simulink library "Lib_LongPRACH"  (R2023b)
settings: Solver=VariableStepAuto  StartTime=0.0  StopTime=10.0  RelTol=1e-3
values from neighbouring files (symbols this model uses):
  prach = waveconfig.PRACH.Config    [hNRPRACHWaveformGenerator.m]
undefined symbols (not defined in the file or in its folder): AdvDSPBChannelOutDisplay, AdvDSPBDMemDisplay, AdvDSPBInDisplay, AdvDSPBOutDisplay, dpoly, dspba, dspba_ChannelInVis, dspba_ChannelOutVis, dspba_internal_get_channel_ports, evalAionMaskParam, latency, latencyCorrection, NTxAnts, primtype, UseDontCare, value
libraries: DSPBAPrim x553, DSPBABase x32, DSPBAFilters x24, DSPBAControl x18, DSPBAModelBus x8, DSPBAWaveformSynth x4, DspbAdvFftLibrary x2, DSPBAUtilities x2
(part 6 of 8)

== system Lib_LongPRACH/prach_wrap/SYM_SELECT/Zero_insertion/Zeropad_rear ==
  valid_in : Inport
  chin : Inport  Port=2
  datain : Inport  Port=3
  And : DSPBAPrim/And  primtype=and  nInputs=2  nOutputs=1  omode=Inherit via internal rule  otype=sfix(16)  scale=2^-15  rndmethod=Unbiased  factor=1  satmethod=Symmetric  shift_vec=[0 1 2 -1]  value=0  inPortNames=[' '; ' '; ' '; ' '; ' '; ' '; ' '; ' '; ' '; ' '; ' '; ' '; ' '; ' '; ' '; ' '; ]  outPortNames=[' ']  dspbaimage=dspba_prim.svg  text=fprintf('&');  style=Optimised  visibilities=8+2  version=20211007
  Const3 : DSPBAPrim/Const  primtype=const  nInputs=0  nOutputs=1  omode=Inherit via internal rule  otype=sfix(16)  scale=2^-15  rndmethod=Unbiased  factor=1  satmethod=Symmetric  shift_vec=[0 1 2 -1]  value=0  inPortNames=['+'; '+';]  outPortNames=[' ']  dspbaimage=dspba_prim.svg  text=fprintf('%s', num2str(value));  style=Optimised  visibilities=8 + 1024 + 2^18 + 2^20  floatPrecision=float32_m23  warnSaturation=on  version=20211007  SampleTime=inf
  Mux1 : DSPBAPrim/Mux  primtype=mux  nInputs=evalAionMaskParam(gcb,'value',1)+1  nOutputs=1  omode=Inherit via internal rule  otype=sfix(16)  scale=2^-15  rndmethod=Unbiased  factor=1  satmethod=Symmetric  shift_vec=[0 1 2 -1]  value=2  inPortNames=['s '; 'd0'; 'd1'; 'd2'; 'd3'; 'd4'; 'd5'; 'd6'; 'd7'; 'd8'; 'd9';]  outPortNames=[' ']  dspbaimage=dspba_prim_tall.svg  text=fprintf('%s', primtype);  style=Optimised  visibilities=1032  version=20211007
  Not : DSPBAPrim/Not  primtype=not  nInputs=1  nOutputs=1  omode=Inherit via internal rule  otype=sfix(16)  scale=2^-15  rndmethod=Unbiased  factor=1  satmethod=Symmetric  shift_vec=[0 1 2 -1]  value=0  inPortNames=[' '; ' ';]  outPortNames=[' ']  dspbaimage=dspba_prim.svg  text=fprintf('~');  style=Optimised  visibilities=8  version=20211007
  Or : DSPBAPrim/Or  primtype=or  nInputs=2  nOutputs=1  omode=Inherit via internal rule  otype=sfix(16)  scale=2^-15  rndmethod=Unbiased  factor=1  satmethod=Symmetric  shift_vec=[0 1 2 -1]  value=0  inPortNames=[' '; ' '; ' '; ' '; ' '; ' '; ' '; ' '; ' '; ' '; ' '; ' '; ' '; ' '; ' '; ' '; ]  outPortNames=[' ']  dspbaimage=dspba_prim.svg  text=fprintf('|');  style=Optimised  visibilities=8+2  version=20211007
  SampleDelay2 : DSPBAPrim/SampleDelay  primtype=sampdelay  nInputs=1  nOutputs=1  omode=Inherit via internal rule  otype=sfix(16)  scale=2^-15  rndmethod=Unbiased  factor=1  satmethod=Symmetric  shift_vec=[0 1 2 -1]  floatPrecision=float32_m23  value=ZeroPadRear  inPortNames=[' '; ' ';]  outPortNames=[' ']  dspbaimage=dspba_prim.svg  text=dpoly(1, eye(1,value+1), 'z')  style=Optimised  visibilities=8 + 2^11 + 2^18 + 2^19  flexible=off  slackgroup=0  augmented=0  version=20211007  advOptions=[]
  valid_out : Outport
  "chout " : Outport  Port=2
  dataout : Outport  Port=3
  wires:
  Const3/1 -> Mux1/3
  Mux1/1 -> dataout/1
  Not/1 -> And/2
  Or/1 -> valid_out/1
  datain/1 -> Mux1/2
  chin/1 -> "chout "/1
  SampleDelay2/1 -> And/1, Or/2
  valid_in/1 -> Not/1, Or/1, SampleDelay2/1
  And/1 -> Mux1/1

== system Lib_LongPRACH/Longprach_C_M_plane/LongPRACH_core/CP_REMOVAL/RemoveCP5/syncgen ==
  In1 : Inport
  CmpEQ : DSPBAPrim/CmpEQ  primtype=cmpeq  nInputs=2  nOutputs=1  omode=boolean  otype=sfix(16)  scale=2^-15  rndmethod=Unbiased  factor=1  satmethod=Symmetric  shift_vec=[0 1 2 -1]  value=0  inPortNames=[' '; ' ';]  outPortNames=[' ']  dspbaimage=dspba_prim.svg  text=fprintf('==');  style=Optimised  visibilities=0  advOptions=[]  version=20211007
  Const2 : DSPBAPrim/Const  primtype=const  nInputs=0  nOutputs=1  omode=Inherit via internal rule  otype=sfix(16)  scale=2^-15  rndmethod=Unbiased  factor=1  satmethod=Symmetric  shift_vec=[0 1 2 -1]  value=10  inPortNames=['+'; '+';]  outPortNames=[' ']  dspbaimage=dspba_prim.svg  text=fprintf('%s', num2str(value));  style=Optimised  visibilities=8 + 1024 + 2^18 + 2^20  floatPrecision=float32_m23  warnSaturation=on  version=20211007  SampleTime=inf
  Const3 : DSPBAPrim/Const  primtype=const  nInputs=0  nOutputs=1  omode=Inherit via internal rule  otype=sfix(16)  scale=2^-15  rndmethod=Unbiased  factor=1  satmethod=Symmetric  shift_vec=[0 1 2 -1]  value=4  inPortNames=['+'; '+';]  outPortNames=[' ']  dspbaimage=dspba_prim.svg  text=fprintf('%s', num2str(value));  style=Optimised  visibilities=8 + 1024 + 2^18 + 2^20  floatPrecision=float32_m23  warnSaturation=on  version=20211007  SampleTime=inf
  StretchPulse : DSPBAControl/StretchPulse
  q : Outport
  wires:
  Const2/1 -> CmpEQ/2
  CmpEQ/1 -> StretchPulse/1
  Const3/1 -> StretchPulse/2
  StretchPulse/1 -> q/1
  In1/1 -> CmpEQ/1

== system Lib_LongPRACH/Longprach_C_M_plane/LongPRACH_core/DECIMATION1/Stage1/Filt_DEC_by_3_stage1 ==
  din : Inport
  vin : Inport  Port=2
  cin : Inport  Port=3
  Complex to Real-Imag : ComplexToRealImag
  Const1 : DSPBAPrim/Const  primtype=const  nInputs=0  nOutputs=1  omode=Inherit via back propagation  otype=ufix(8)  scale=2^0  rndmethod=Unbiased  factor=1  satmethod=Symmetric  shift_vec=[0 1 2 -1]  value=deimator_shift  inPortNames=['+'; '+';]  outPortNames=[' ']  dspbaimage=dspba_prim.svg  text=fprintf('%s', num2str(value));  style=Optimised  visibilities=8 + 1024  floatPrecision=float32_m23  warnSaturation=on  version=20211007  SampleTime=inf
  Const6 : DSPBAPrim/Const  primtype=const  nInputs=0  nOutputs=1  omode=Inherit via back propagation  otype=ufix(8)  scale=2^0  rndmethod=Unbiased  factor=1  satmethod=Symmetric  shift_vec=[0 1 2 -1]  value=deimator_shift  inPortNames=['+'; '+';]  outPortNames=[' ']  dspbaimage=dspba_prim.svg  text=fprintf('%s', num2str(value));  style=Optimised  visibilities=8 + 1024  floatPrecision=float32_m23  warnSaturation=on  version=20211007  SampleTime=inf
  DecimatingFIR1 : DSPBAFilters/DecimatingFIR  nInputRate=prach.MaxSampleRate  decim=3  nchan=prach.no_of_chan  symmetry=Symmetrical  coef=b_decimator1  addr=MMoffset.decby3_st2  rwmode=Constant  nband=Use All Taps  exposebus=off  latency=26  version=20090407  recon=off  MM=[0,1,2,3,4,5,6,7,8,9,10,11,12,13,14,15]  resetrezero=off  sharecoef=auto  simulationMode=Standard
  DecimatingFIR2 : DSPBAFilters/DecimatingFIR  nInputRate=prach.MaxSampleRate  decim=3  nchan=prach.no_of_chan  symmetry=Symmetrical  coef=b_decimator1  addr=MMoffset.decby3_st2  rwmode=Constant  nband=Use All Taps  exposebus=off  latency=26  version=20090407  recon=off  MM=[0,1,2,3,4,5,6,7,8,9,10,11,12,13,14,15]  resetrezero=off  sharecoef=auto  simulationMode=Standard
  Real-Imag to Complex : RealImagToComplex
  Scale : DSPBABase/Scale  otype=sfix(16)  scale=2^-15  rndmethod=Biased  factor=decimator_gain1  satmethod=Symmetric  shift_vec=0  latency=5  simulationMode=Use Global Value  version=20130807
  Scale1 : DSPBABase/Scale  otype=sfix(16)  scale=2^-15  rndmethod=Biased  factor=decimator_gain1  satmethod=Symmetric  shift_vec=0  latency=5  simulationMode=Use Global Value  version=20130807
  Terminator : Terminator
  Terminator1 : Terminator
  To Workspace3 : ToWorkspace  VariableName=dec_dout_stage1  SampleTime=-1
  To Workspace4 : ToWorkspace  VariableName=dec_vout_stage1  SampleTime=-1
  dout : Outport  VectorParamsAs1DForOutWhenUnconnected=off
  vout : Outport  Port=2  VectorParamsAs1DForOutWhenUnconnected=off
  cout : Outport  Port=3  VectorParamsAs1DForOutWhenUnconnected=off
  wires:
  Scale/3 -> cout/1
  DecimatingFIR2/2 -> Scale/2
  vin/1 -> DecimatingFIR1/2, DecimatingFIR2/2
  DecimatingFIR2/3 -> Scale/3
  Scale/2 -> To Workspace4/1, vout/1
  Scale/4 -> Terminator/1
  cin/1 -> DecimatingFIR1/3, DecimatingFIR2/3
  Const6/1 -> Scale/4
  DecimatingFIR2/1 -> Scale/1
  din/1 -> Complex to Real-Imag/1
  Complex to Real-Imag/1 -> DecimatingFIR2/1
  Complex to Real-Imag/2 -> DecimatingFIR1/1
  Scale1/1 -> Real-Imag to Complex/2
  DecimatingFIR1/3 -> Scale1/3
  Scale1/4 -> Terminator1/1
  DecimatingFIR1/1 -> Scale1/1
  DecimatingFIR1/2 -> Scale1/2
  Const1/1 -> Scale1/4
  Real-Imag to Complex/1 -> To Workspace3/1, dout/1
  Scale/1 -> Real-Imag to Complex/1

== system Lib_LongPRACH/Longprach_C_M_plane/LongPRACH_core/DECIMATION1/Stage1/filt_flush_in ==
  note: 1 0 0 0
  data_in : Inport
  valid_in : Inport  Port=2
  ch_in : Inport  Port=3
  flush_en : Inport  Port=4
  ChannelIn : DSPBAPrim/ChannelIn  primtype=channelin  nInputs=dspba_internal_get_channel_ports(gcb)  nOutputs=dspba_internal_get_channel_ports(gcb)  omode=Inherit via internal rule  otype=sfix(16)  scale=2^-15  rndmethod=Unbiased  factor=1  satmethod=Symmetric  shift_vec=[0 1 2 -1]  value=2  inPortNames=['v'; 'c'; '0'; '1'; '2'; '3'; '4'; '5'; '6'; '7'; '8'; '9'; 'A'; 'B'; 'D'; 'E'; 'F'; 'G'; 'H'; 'I'; 'J'; 'K'; 'L'; 'M'; 'N'; 'O'; 'P'; 'Q'; 'R'; 'S'; 'T'; 'U'; 'W'; 'X'; 'Y'; 'Z']  outPortNames=['v'; 'c'; '0'; '1'; '2'; '3'; '4'; '5'; '6'; '7'; '8'; '9'; 'A'; 'B'; 'D'; 'E'; 'F'; 'G'; 'H'; 'I'; 'J'; 'K'; 'L'; 'M'; 'N'; 'O'; 'P'; 'Q'; 'R'; 'S'; 'T'; 'U'; 'W'; 'X'; 'Y'; 'Z']  dspbaimage=dspba_prim_channel_tall.svg  text=fprintf('In');  style=Optimised  dataSignals=2  foldingEnabled=off  channels=1  sampleRate=200  packetBeginPresent=off  packetBeginEnabled=off  visibilities=dspba_ChannelInVis(gcb)  latencyCorrection=0  scheduleOrigin=on  version=20211214
  ChannelOut : DSPBAPrim/ChannelOut  primtype=channelout  nInputs=dspba_internal_get_channel_ports(gcb)  nOutputs=dspba_internal_get_channel_ports(gcb)  omode=Inherit via internal rule  otype=sfix(16)  scale=2^-15  rndmethod=Unbiased  factor=1  satmethod=Symmetric  shift_vec=[0 1 2 -1]  value=1  inPortNames=['v'; 'c'; '0'; '1'; '2'; '3'; '4'; '5'; '6'; '7'; '8'; '9'; 'A'; 'B'; 'D'; 'E'; 'F'; 'G'; 'H'; 'I'; 'J'; 'K'; 'L'; 'M'; 'N'; 'O'; 'P'; 'Q'; 'R'; 'S'; 'T'; 'U'; 'W'; 'X'; 'Y'; 'Z']  outPortNames=['v'; 'c'; '0'; '1'; '2'; '3'; '4'; '5'; '6'; '7'; '8'; '9'; 'A'; 'B'; 'D'; 'E'; 'F'; 'G'; 'H'; 'I'; 'J'; 'K'; 'L'; 'M'; 'N'; 'O'; 'P'; 'Q'; 'R'; 'S'; 'T'; 'U'; 'W'; 'X'; 'Y'; 'Z']  dspbaimage=dspba_prim_channel_tall.svg  text=fprintf('Out%s', AdvDSPBChannelOutDisplay(latency));  style=Optimised  dataSignals=1  foldingEnabled=off  channels=1  sampleRate=200  packetBeginPresent=off  packetBeginEnabled=off  visibilities=dspba_ChannelOutVis(gcb)  latency=1  latencyCorrection=0  version=20211214
  Const1 : DSPBAPrim/Const  primtype=const  nInputs=0  nOutputs=1  omode=Inherit via internal rule  otype=sfix(16)  scale=2^-15  rndmethod=Unbiased  factor=1  satmethod=Symmetric  shift_vec=[0 1 2 -1]  value=0  inPortNames=['+'; '+';]  outPortNames=[' ']  dspbaimage=dspba_prim.svg  text=fprintf('%s', num2str(value));  style=Optimised  visibilities=8 + 1024 + 2^18 + 2^20  floatPrecision=float32_m23  warnSaturation=on  version=20211007  SampleTime=inf
  Mux : DSPBAPrim/Mux  primtype=mux  nInputs=evalAionMaskParam(gcb,'value',1)+1  nOutputs=1  omode=Inherit via internal rule  otype=sfix(16)  scale=2^-15  rndmethod=Unbiased  factor=1  satmethod=Symmetric  shift_vec=[0 1 2 -1]  value=2  inPortNames=['s '; 'd0'; 'd1'; 'd2'; 'd3'; 'd4'; 'd5'; 'd6'; 'd7'; 'd8'; 'd9';]  outPortNames=[' ']  dspbaimage=dspba_prim_tall.svg  text=fprintf('%s', primtype);  style=Optimised  visibilities=1032  version=20211007
  Mux1 : DSPBAPrim/Mux  primtype=mux  nInputs=evalAionMaskParam(gcb,'value',1)+1  nOutputs=1  omode=Inherit via internal rule  otype=sfix(16)  scale=2^-15  rndmethod=Unbiased  factor=1  satmethod=Symmetric  shift_vec=[0 1 2 -1]  value=2  inPortNames=['s '; 'd0'; 'd1'; 'd2'; 'd3'; 'd4'; 'd5'; 'd6'; 'd7'; 'd8'; 'd9';]  outPortNames=[' ']  dspbaimage=dspba_prim_tall.svg  text=fprintf('%s', primtype);  style=Optimised  visibilities=1032  version=20211007
  Mux2 : DSPBAPrim/Mux  primtype=mux  nInputs=evalAionMaskParam(gcb,'value',1)+1  nOutputs=1  omode=Inherit via internal rule  otype=sfix(16)  scale=2^-15  rndmethod=Unbiased  factor=1  satmethod=Symmetric  shift_vec=[0 1 2 -1]  value=2  inPortNames=['s '; 'd0'; 'd1'; 'd2'; 'd3'; 'd4'; 'd5'; 'd6'; 'd7'; 'd8'; 'd9';]  outPortNames=[' ']  dspbaimage=dspba_prim_tall.svg  text=fprintf('%s', primtype);  style=Optimised  visibilities=1032  version=20211007
  SynthesisInfo : DSPBAPrim/SynthesisInfo  primtype=synthinfo  nInputs=0  nOutputs=0  omode=Inherit via internal rule  otype=sfix(16)  scale=2^-15  rndmethod=Truncate  factor=1  satmethod=Symmetric  shift_vec=[0 1 2 -1]  value=99  inPortNames=[' '; ' ';]  outPortNames=[' ']  dspbaimage=dspba_prim_ctrl.jpg  text=fprintf('Style=%s', style);  style=Scheduled  visibilities=2^17+2^18+2^19+2^20+2^21+2^22+2^23+2^24  constraintPair=None  constraintRelation=>  constraintLimit=2  modelRefSign=+  modelRef=''  showSchedule=off  simulationMode=Use Global Value  resetMinimization=Conditional - On for ChannelIn/Out only  version=20220106
  ch_pulse : Subsystem
  data_out : Outport
  valid_out : Outport  Port=2
  ch_out : Outport  Port=3
  wires:
  Mux/1 -> ChannelOut/1
  ChannelOut/1 -> valid_out/1
  Mux2/1 -> ChannelOut/3
  flush_en/1 -> ChannelIn/4
  Const1/1 -> Mux2/3
  ChannelOut/3 -> data_out/1
  ChannelIn/2 -> Mux1/2
  ChannelOut/2 -> ch_out/1
  ch_in/1 -> ChannelIn/2
  ChannelIn/1 -> Mux/2
  valid_in/1 -> ChannelIn/1
  ChannelIn/3 -> Mux2/2
  ChannelIn/4 -> Mux2/1, ch_pulse/1(In1), Mux1/1, Mux/1, Mux/3
  Mux1/1 -> ChannelOut/2
  data_in/1 -> ChannelIn/3
  ch_pulse/1(Out1) -> Mux1/3

== system Lib_LongPRACH/Longprach_C_M_plane/LongPRACH_core/DECIMATION1/Stage2/Filt_DEC_by_2_stage2 ==
  din : Inport
  vin : Inport  Port=2
  cin : Inport  Port=3
  Complex to Real-Imag : ComplexToRealImag
  Const1 : DSPBAPrim/Const  primtype=const  nInputs=0  nOutputs=1  omode=Inherit via back propagation  otype=ufix(8)  scale=2^0  rndmethod=Unbiased  factor=1  satmethod=Symmetric  shift_vec=[0 1 2 -1]  value=deimator_shift  inPortNames=['+'; '+';]  outPortNames=[' ']  dspbaimage=dspba_prim.svg  text=fprintf('%s', num2str(value));  style=Optimised  visibilities=8 + 1024  floatPrecision=float32_m23  warnSaturation=on  version=20211007  SampleTime=inf
  Const6 : DSPBAPrim/Const  primtype=const  nInputs=0  nOutputs=1  omode=Inherit via back propagation  otype=ufix(8)  scale=2^0  rndmethod=Unbiased  factor=1  satmethod=Symmetric  shift_vec=[0 1 2 -1]  value=deimator_shift  inPortNames=['+'; '+';]  outPortNames=[' ']  dspbaimage=dspba_prim.svg  text=fprintf('%s', num2str(value));  style=Optimised  visibilities=8 + 1024  floatPrecision=float32_m23  warnSaturation=on  version=20211007  SampleTime=inf
  DecimatingFIR : DSPBAFilters/DecimatingFIR  nInputRate=prach.MaxSampleRate/3  decim=2  nchan=prach.no_of_chan  symmetry=Symmetrical  coef=b_decimator2  addr=MMoffset.HBcoef3  rwmode=Constant  nband=Use All Taps  exposebus=off  latency=34  version=20090407  recon=off  MM=[0,1,2,3,4,5,6,7,8,9,10,11,12,13,14,15]  resetrezero=off  sharecoef=auto  simulationMode=Standard
  DecimatingFIR1 : DSPBAFilters/DecimatingFIR  nInputRate=prach.MaxSampleRate/3  decim=2  nchan=prach.no_of_chan  symmetry=Symmetrical  coef=b_decimator2  addr=MMoffset.HBcoef3  rwmode=Constant  nband=Use All Taps  exposebus=off  latency=34  version=20090407  recon=off  MM=[0,1,2,3,4,5,6,7,8,9,10,11,12,13,14,15]  resetrezero=off  sharecoef=auto  simulationMode=Standard
  Real-Imag to Complex : RealImagToComplex
  Scale : DSPBABase/Scale  otype=sfix(16)  scale=2^-15  rndmethod=Biased  factor=decimator_gain2  satmethod=Symmetric  shift_vec=0  latency=5  simulationMode=Use Global Value  version=20130807
  Scale1 : DSPBABase/Scale  otype=sfix(16)  scale=2^-15  rndmethod=Biased  factor=decimator_gain2  satmethod=Symmetric  shift_vec=0  latency=5  simulationMode=Use Global Value  version=20130807
  Terminator{,1..3} (4 alike) : Terminator
  To Workspace3 : ToWorkspace  VariableName=dec_dout_stage2  SampleTime=-1
  To Workspace4 : ToWorkspace  VariableName=dec_vout_stage2  SampleTime=-1
  dout : Outport  VectorParamsAs1DForOutWhenUnconnected=off
  vout : Outport  Port=2  VectorParamsAs1DForOutWhenUnconnected=off
  cout : Outport  Port=3  VectorParamsAs1DForOutWhenUnconnected=off
  wires:
  DecimatingFIR/1 -> Scale/1
  Const6/1 -> Scale/4
  cin/1 -> DecimatingFIR1/3, DecimatingFIR/3
  Scale/4 -> Terminator/1
  DecimatingFIR/3 -> Scale/3
  vin/1 -> DecimatingFIR1/2, DecimatingFIR/2
  DecimatingFIR/2 -> Scale/2
  Scale/3 -> cout/1
  din/1 -> Complex to Real-Imag/1
  Complex to Real-Imag/1 -> DecimatingFIR/1
  Complex to Real-Imag/2 -> DecimatingFIR1/1
  DecimatingFIR1/1 -> Scale1/1
  DecimatingFIR1/3 -> Scale1/3
  Scale1/1 -> Real-Imag to Complex/2
  DecimatingFIR1/2 -> Scale1/2
  Const1/1 -> Scale1/4
  Scale1/4 -> Terminator1/1
  Scale/1 -> Real-Imag to Complex/1
  Scale1/2 -> Terminator2/1
  Scale1/3 -> Terminator3/1
  Scale/2 -> To Workspace4/1, vout/1
  Real-Imag to Complex/1 -> To Workspace3/1, dout/1

== system Lib_LongPRACH/Longprach_C_M_plane/LongPRACH_core/DECIMATION1/Stage3/Filt_DEC_by_2_stage3 ==
  din : Inport
  vin : Inport  Port=2
  cin : Inport  Port=3
  Complex to Real-Imag : ComplexToRealImag
  Const1 : DSPBAPrim/Const  primtype=const  nInputs=0  nOutputs=1  omode=Inherit via back propagation  otype=ufix(8)  scale=2^0  rndmethod=Unbiased  factor=1  satmethod=Symmetric  shift_vec=[0 1 2 -1]  value=deimator_shift  inPortNames=['+'; '+';]  outPortNames=[' ']  dspbaimage=dspba_prim.svg  text=fprintf('%s', num2str(value));  style=Optimised  visibilities=8 + 1024  floatPrecision=float32_m23  warnSaturation=on  version=20211007  SampleTime=inf
  Const6 : DSPBAPrim/Const  primtype=const  nInputs=0  nOutputs=1  omode=Inherit via back propagation  otype=ufix(8)  scale=2^0  rndmethod=Unbiased  factor=1  satmethod=Symmetric  shift_vec=[0 1 2 -1]  value=deimator_shift  inPortNames=['+'; '+';]  outPortNames=[' ']  dspbaimage=dspba_prim.svg  text=fprintf('%s', num2str(value));  style=Optimised  visibilities=8 + 1024  floatPrecision=float32_m23  warnSaturation=on  version=20211007  SampleTime=inf
  DecimatingFIR : DSPBAFilters/DecimatingFIR  nInputRate=prach.MaxSampleRate/(3*2)  decim=2  nchan=prach.no_of_chan  symmetry=Symmetrical  coef=b_decimator3  addr=MMoffset.HBcoef3  rwmode=Constant  nband=Use All Taps  exposebus=off  latency=46  version=20090407  recon=off  MM=[0,1,2,3,4,5,6,7,8,9,10,11,12,13,14,15]  resetrezero=off  sharecoef=auto  simulationMode=Standard
  DecimatingFIR1 : DSPBAFilters/DecimatingFIR  nInputRate=prach.MaxSampleRate/(3*2)  decim=2  nchan=prach.no_of_chan  symmetry=Symmetrical  coef=b_decimator3  addr=MMoffset.HBcoef3  rwmode=Constant  nband=Use All Taps  exposebus=off  latency=46  version=20090407  recon=off  MM=[0,1,2,3,4,5,6,7,8,9,10,11,12,13,14,15]  resetrezero=off  sharecoef=auto  simulationMode=Standard
  Real-Imag to Complex : RealImagToComplex
  Scale : DSPBABase/Scale  otype=sfix(16)  scale=2^-15  rndmethod=Biased  factor=decimator_gain3  satmethod=Symmetric  shift_vec=0  latency=5  simulationMode=Use Global Value  version=20130807
  Scale1 : DSPBABase/Scale  otype=sfix(16)  scale=2^-15  rndmethod=Biased  factor=decimator_gain3  satmethod=Symmetric  shift_vec=0  latency=5  simulationMode=Use Global Value  version=20130807
  Terminator{,1..3} (4 alike) : Terminator
  To Workspace3 : ToWorkspace  VariableName=dec_dout_stage3  SampleTime=-1
  To Workspace4 : ToWorkspace  VariableName=dec_vout_stage3  SampleTime=-1
  dout : Outport  VectorParamsAs1DForOutWhenUnconnected=off
  vout : Outport  Port=2  VectorParamsAs1DForOutWhenUnconnected=off
  cout : Outport  Port=3  VectorParamsAs1DForOutWhenUnconnected=off
  wires:
  DecimatingFIR/1 -> Scale/1
  Const6/1 -> Scale/4
  cin/1 -> DecimatingFIR1/3, DecimatingFIR/3
  Scale/4 -> Terminator/1
  DecimatingFIR/3 -> Scale/3
  vin/1 -> DecimatingFIR1/2, DecimatingFIR/2
  DecimatingFIR/2 -> Scale/2
  Scale/3 -> cout/1
  din/1 -> Complex to Real-Imag/1
  Complex to Real-Imag/1 -> DecimatingFIR/1
  Complex to Real-Imag/2 -> DecimatingFIR1/1
  DecimatingFIR1/1 -> Scale1/1
  DecimatingFIR1/3 -> Scale1/3
  Scale1/1 -> Real-Imag to Complex/2
  DecimatingFIR1/2 -> Scale1/2
  Const1/1 -> Scale1/4
  Scale1/4 -> Terminator1/1
  Scale/1 -> Real-Imag to Complex/1
  Scale1/2 -> Terminator2/1
  Scale1/3 -> Terminator3/1
  Scale/2 -> To Workspace4/1, vout/1
  Real-Imag to Complex/1 -> To Workspace3/1, dout/1

== system Lib_LongPRACH/Longprach_C_M_plane/LongPRACH_core/DECIMATION1/Stage5/Filt_DEC_by_2_stage5 ==
  din : Inport
  vin : Inport  Port=2
  cin : Inport  Port=3
  Complex to Real-Imag : ComplexToRealImag
  Const1 : DSPBAPrim/Const  primtype=const  nInputs=0  nOutputs=1  omode=Inherit via back propagation  otype=ufix(8)  scale=2^0  rndmethod=Unbiased  factor=1  satmethod=Symmetric  shift_vec=[0 1 2 -1]  value=deimator_shift  inPortNames=['+'; '+';]  outPortNames=[' ']  dspbaimage=dspba_prim.svg  text=fprintf('%s', num2str(value));  style=Optimised  visibilities=8 + 1024  floatPrecision=float32_m23  warnSaturation=on  version=20211007  SampleTime=inf
  Const6 : DSPBAPrim/Const  primtype=const  nInputs=0  nOutputs=1  omode=Inherit via back propagation  otype=ufix(8)  scale=2^0  rndmethod=Unbiased  factor=1  satmethod=Symmetric  shift_vec=[0 1 2 -1]  value=deimator_shift  inPortNames=['+'; '+';]  outPortNames=[' ']  dspbaimage=dspba_prim.svg  text=fprintf('%s', num2str(value));  style=Optimised  visibilities=8 + 1024  floatPrecision=float32_m23  warnSaturation=on  version=20211007  SampleTime=inf
  DecimatingFIR : DSPBAFilters/DecimatingFIR  nInputRate=prach.MaxSampleRate/(3*2*2*2)  decim=2  nchan=prach.no_of_chan  symmetry=Symmetrical  coef=b_decimator5  addr=MMoffset.HBcoef3  rwmode=Constant  nband=Use All Taps  exposebus=off  latency=176  version=20090407  recon=off  MM=[0,1,2,3,4,5,6,7,8,9,10,11,12,13,14,15]  resetrezero=off  sharecoef=auto  simulationMode=Standard
  DecimatingFIR1 : DSPBAFilters/DecimatingFIR  nInputRate=prach.MaxSampleRate/(3*2*2*2)  decim=2  nchan=prach.no_of_chan  symmetry=Symmetrical  coef=b_decimator5  addr=MMoffset.HBcoef3  rwmode=Constant  nband=Use All Taps  exposebus=off  latency=176  version=20090407  recon=off  MM=[0,1,2,3,4,5,6,7,8,9,10,11,12,13,14,15]  resetrezero=off  sharecoef=auto  simulationMode=Standard
  Real-Imag to Complex : RealImagToComplex
  Scale : DSPBABase/Scale  otype=sfix(16)  scale=2^-15  rndmethod=Biased  factor=decimator_gain5  satmethod=Symmetric  shift_vec=0  latency=5  simulationMode=Use Global Value  version=20130807
  Scale1 : DSPBABase/Scale  otype=sfix(16)  scale=2^-15  rndmethod=Biased  factor=decimator_gain5  satmethod=Symmetric  shift_vec=0  latency=5  simulationMode=Use Global Value  version=20130807
  Terminator{,1..3} (4 alike) : Terminator
  To Workspace3 : ToWorkspace  VariableName=dec_dout_stage5  SampleTime=-1
  To Workspace4 : ToWorkspace  VariableName=dec_vout_stage5  SampleTime=-1
  dout : Outport  VectorParamsAs1DForOutWhenUnconnected=off
  vout : Outport  Port=2  VectorParamsAs1DForOutWhenUnconnected=off
  cout : Outport  Port=3  VectorParamsAs1DForOutWhenUnconnected=off
  wires:
  DecimatingFIR/1 -> Scale/1
  Const6/1 -> Scale/4
  cin/1 -> DecimatingFIR1/3, DecimatingFIR/3
  Scale/4 -> Terminator/1
  DecimatingFIR/3 -> Scale/3
  vin/1 -> DecimatingFIR1/2, DecimatingFIR/2
  DecimatingFIR/2 -> Scale/2
  Scale/3 -> cout/1
  din/1 -> Complex to Real-Imag/1
  Complex to Real-Imag/1 -> DecimatingFIR/1
  Complex to Real-Imag/2 -> DecimatingFIR1/1
  DecimatingFIR1/1 -> Scale1/1
  DecimatingFIR1/3 -> Scale1/3
  Scale1/1 -> Real-Imag to Complex/2
  DecimatingFIR1/2 -> Scale1/2
  Const1/1 -> Scale1/4
  Scale1/4 -> Terminator1/1
  Scale/1 -> Real-Imag to Complex/1
  Scale1/2 -> Terminator2/1
  Scale1/3 -> Terminator3/1
  Scale/2 -> vout/1, To Workspace4/1
  Real-Imag to Complex/1 -> dout/1, To Workspace3/1

== system Lib_LongPRACH/Longprach_C_M_plane/LongPRACH_core/DECIMATION1/Stage6/Filt_DEC_by_2_stage6 ==
  din : Inport
  vin : Inport  Port=2
  cin : Inport  Port=3
  Complex to Real-Imag : ComplexToRealImag
  Const1 : DSPBAPrim/Const  primtype=const  nInputs=0  nOutputs=1  omode=Inherit via back propagation  otype=ufix(8)  scale=2^0  rndmethod=Unbiased  factor=1  satmethod=Symmetric  shift_vec=[0 1 2 -1]  value=deimator_shift  inPortNames=['+'; '+';]  outPortNames=[' ']  dspbaimage=dspba_prim.svg  text=fprintf('%s', num2str(value));  style=Optimised  visibilities=8 + 1024  floatPrecision=float32_m23  warnSaturation=on  version=20211007  SampleTime=inf
  Const6 : DSPBAPrim/Const  primtype=const  nInputs=0  nOutputs=1  omode=Inherit via back propagation  otype=ufix(8)  scale=2^0  rndmethod=Unbiased  factor=1  satmethod=Symmetric  shift_vec=[0 1 2 -1]  value=deimator_shift  inPortNames=['+'; '+';]  outPortNames=[' ']  dspbaimage=dspba_prim.svg  text=fprintf('%s', num2str(value));  style=Optimised  visibilities=8 + 1024  floatPrecision=float32_m23  warnSaturation=on  version=20211007  SampleTime=inf
  DecimatingFIR : DSPBAFilters/DecimatingFIR  nInputRate=prach.MaxSampleRate/(3*2*2*2*2)  decim=2  nchan=prach.no_of_chan  symmetry=Symmetrical  coef=b_decimator6  addr=MMoffset.HBcoef3  rwmode=Constant  nband=Use All Taps  exposebus=off  latency=208  version=20090407  recon=off  MM=[0,1,2,3,4,5,6,7,8,9,10,11,12,13,14,15]  resetrezero=off  sharecoef=auto  simulationMode=Standard
  DecimatingFIR1 : DSPBAFilters/DecimatingFIR  nInputRate=prach.MaxSampleRate/(3*2*2*2*2)  decim=2  nchan=prach.no_of_chan  symmetry=Symmetrical  coef=b_decimator6  addr=MMoffset.HBcoef3  rwmode=Constant  nband=Use All Taps  exposebus=off  latency=208  version=20090407  recon=off  MM=[0,1,2,3,4,5,6,7,8,9,10,11,12,13,14,15]  resetrezero=off  sharecoef=auto  simulationMode=Standard
  Real-Imag to Complex : RealImagToComplex
  Scale : DSPBABase/Scale  otype=sfix(16)  scale=2^-15  rndmethod=Biased  factor=decimator_gain6  satmethod=Symmetric  shift_vec=0  latency=5  simulationMode=Use Global Value  version=20130807
  Scale1 : DSPBABase/Scale  otype=sfix(16)  scale=2^-15  rndmethod=Biased  factor=decimator_gain6  satmethod=Symmetric  shift_vec=0  latency=5  simulationMode=Use Global Value  version=20130807
  Terminator{,1..3} (4 alike) : Terminator
  dout : Outport  VectorParamsAs1DForOutWhenUnconnected=off
  vout : Outport  Port=2  VectorParamsAs1DForOutWhenUnconnected=off
  cout : Outport  Port=3  VectorParamsAs1DForOutWhenUnconnected=off
  wires:
  DecimatingFIR/1 -> Scale/1
  Const6/1 -> Scale/4
  cin/1 -> DecimatingFIR1/3, DecimatingFIR/3
  Scale/4 -> Terminator/1
  Scale/2 -> vout/1
  DecimatingFIR/3 -> Scale/3
  vin/1 -> DecimatingFIR1/2, DecimatingFIR/2
  DecimatingFIR/2 -> Scale/2
  Scale/3 -> cout/1
  din/1 -> Complex to Real-Imag/1
  Complex to Real-Imag/1 -> DecimatingFIR/1
  Complex to Real-Imag/2 -> DecimatingFIR1/1
  DecimatingFIR1/1 -> Scale1/1
  DecimatingFIR1/3 -> Scale1/3
  Scale1/1 -> Real-Imag to Complex/2
  DecimatingFIR1/2 -> Scale1/2
  Const1/1 -> Scale1/4
  Scale1/4 -> Terminator1/1
  Scale/1 -> Real-Imag to Complex/1
  Real-Imag to Complex/1 -> dout/1
  Scale1/2 -> Terminator2/1
  Scale1/3 -> Terminator3/1

== system Lib_LongPRACH/Longprach_C_M_plane/LongPRACH_core/DECIMATION1/Stage6/filt_flush_out ==
  data_in : Inport
  valid_in : Inport  Port=2
  ch_in : Inport  Port=3
  flush_en : Inport  Port=4
  ChannelIn : DSPBAPrim/ChannelIn  primtype=channelin  nInputs=dspba_internal_get_channel_ports(gcb)  nOutputs=dspba_internal_get_channel_ports(gcb)  omode=Inherit via internal rule  otype=sfix(16)  scale=2^-15  rndmethod=Unbiased  factor=1  satmethod=Symmetric  shift_vec=[0 1 2 -1]  value=2  inPortNames=['v'; 'c'; '0'; '1'; '2'; '3'; '4'; '5'; '6'; '7'; '8'; '9'; 'A'; 'B'; 'D'; 'E'; 'F'; 'G'; 'H'; 'I'; 'J'; 'K'; 'L'; 'M'; 'N'; 'O'; 'P'; 'Q'; 'R'; 'S'; 'T'; 'U'; 'W'; 'X'; 'Y'; 'Z']  outPortNames=['v'; 'c'; '0'; '1'; '2'; '3'; '4'; '5'; '6'; '7'; '8'; '9'; 'A'; 'B'; 'D'; 'E'; 'F'; 'G'; 'H'; 'I'; 'J'; 'K'; 'L'; 'M'; 'N'; 'O'; 'P'; 'Q'; 'R'; 'S'; 'T'; 'U'; 'W'; 'X'; 'Y'; 'Z']  dspbaimage=dspba_prim_channel_tall.svg  text=fprintf('In');  style=Optimised  dataSignals=2  foldingEnabled=off  channels=1  sampleRate=200  packetBeginPresent=off  packetBeginEnabled=off  visibilities=dspba_ChannelInVis(gcb)  latencyCorrection=0  scheduleOrigin=on  version=20211214
  ChannelOut : DSPBAPrim/ChannelOut  primtype=channelout  nInputs=dspba_internal_get_channel_ports(gcb)  nOutputs=dspba_internal_get_channel_ports(gcb)  omode=Inherit via internal rule  otype=sfix(16)  scale=2^-15  rndmethod=Unbiased  factor=1  satmethod=Symmetric  shift_vec=[0 1 2 -1]  value=1  inPortNames=['v'; 'c'; '0'; '1'; '2'; '3'; '4'; '5'; '6'; '7'; '8'; '9'; 'A'; 'B'; 'D'; 'E'; 'F'; 'G'; 'H'; 'I'; 'J'; 'K'; 'L'; 'M'; 'N'; 'O'; 'P'; 'Q'; 'R'; 'S'; 'T'; 'U'; 'W'; 'X'; 'Y'; 'Z']  outPortNames=['v'; 'c'; '0'; '1'; '2'; '3'; '4'; '5'; '6'; '7'; '8'; '9'; 'A'; 'B'; 'D'; 'E'; 'F'; 'G'; 'H'; 'I'; 'J'; 'K'; 'L'; 'M'; 'N'; 'O'; 'P'; 'Q'; 'R'; 'S'; 'T'; 'U'; 'W'; 'X'; 'Y'; 'Z']  dspbaimage=dspba_prim_channel_tall.svg  text=fprintf('Out%s', AdvDSPBChannelOutDisplay(latency));  style=Optimised  dataSignals=1  foldingEnabled=off  channels=1  sampleRate=200  packetBeginPresent=off  packetBeginEnabled=off  visibilities=dspba_ChannelOutVis(gcb)  latency=1  latencyCorrection=0  version=20211214
  Const : DSPBAPrim/Const  primtype=const  nInputs=0  nOutputs=1  omode=boolean  otype=sfix(16)  scale=2^-15  rndmethod=Unbiased  factor=1  satmethod=Symmetric  shift_vec=[0 1 2 -1]  value=0  inPortNames=['+'; '+';]  outPortNames=[' ']  dspbaimage=dspba_prim.svg  text=fprintf('%s', num2str(value));  style=Optimised  visibilities=8 + 1024 + 2^18 + 2^20  floatPrecision=float32_m23  warnSaturation=on  version=20211007  SampleTime=inf
  Const1 : DSPBAPrim/Const  primtype=const  nInputs=0  nOutputs=1  omode=boolean  otype=sfix(16)  scale=2^-15  rndmethod=Unbiased  factor=1  satmethod=Symmetric  shift_vec=[0 1 2 -1]  value=1  inPortNames=['+'; '+';]  outPortNames=[' ']  dspbaimage=dspba_prim.svg  text=fprintf('%s', num2str(value));  style=Optimised  visibilities=8 + 1024 + 2^18 + 2^20  floatPrecision=float32_m23  warnSaturation=on  version=20211007  SampleTime=inf
  Const2 : DSPBAPrim/Const  primtype=const  nInputs=0  nOutputs=1  omode=Inherit via internal rule  otype=sfix(16)  scale=2^-15  rndmethod=Unbiased  factor=1  satmethod=Symmetric  shift_vec=[0 1 2 -1]  value=filt_flush_hold  inPortNames=['+'; '+';]  outPortNames=[' ']  dspbaimage=dspba_prim.svg  text=fprintf('%s', num2str(value));  style=Optimised  visibilities=8 + 1024 + 2^18 + 2^20  floatPrecision=float32_m23  warnSaturation=on  version=20211007  SampleTime=inf
  Fallingedge : Subsystem
  Loop : DSPBAPrim/Loop  primtype=loop  nInputs=3  nOutputs=4  omode=Inherit via internal rule  otype=sfix(16)  scale=2^-15  rndmethod=Unbiased  factor=1  satmethod=Symmetric  shift_vec=[0 1 2 -1]  value=[zeros(16, 1)]  inPortNames=['g'; 'c'; 'e']  outPortNames=['v'; 'q'; 'f'; 'l']  dspbaimage=dspba_prim_tall.svg  text=fprintf('loop');  style=Optimised  visibilities=0  version=20211007
  Mux : DSPBAPrim/Mux  primtype=mux  nInputs=evalAionMaskParam(gcb,'value',1)+1  nOutputs=1  omode=Inherit via internal rule  otype=sfix(16)  scale=2^-15  rndmethod=Unbiased  factor=1  satmethod=Symmetric  shift_vec=[0 1 2 -1]  value=2  inPortNames=['s '; 'd0'; 'd1'; 'd2'; 'd3'; 'd4'; 'd5'; 'd6'; 'd7'; 'd8'; 'd9';]  outPortNames=[' ']  dspbaimage=dspba_prim_tall.svg  text=fprintf('%s', primtype);  style=Optimised  visibilities=1032  version=20211007
  Or : DSPBAPrim/Or  primtype=or  nInputs=3  nOutputs=1  omode=Inherit via internal rule  otype=sfix(16)  scale=2^-15  rndmethod=Unbiased  factor=1  satmethod=Symmetric  shift_vec=[0 1 2 -1]  value=0  inPortNames=[' '; ' '; ' '; ' '; ' '; ' '; ' '; ' '; ' '; ' '; ' '; ' '; ' '; ' '; ' '; ' '; ]  outPortNames=[' ']  dspbaimage=dspba_prim.svg  text=fprintf('|');  style=Optimised  visibilities=8+2  version=20211007
  SampleDelay : DSPBAPrim/SampleDelay  primtype=sampdelay  nInputs=1  nOutputs=1  omode=Inherit via internal rule  otype=sfix(16)  scale=2^-15  rndmethod=Unbiased  factor=1  satmethod=Symmetric  shift_vec=[0 1 2 -1]  floatPrecision=float32_m23  value=3  inPortNames=[' '; ' ';]  outPortNames=[' ']  dspbaimage=dspba_prim.svg  text=dpoly(1, eye(1,value+1), 'z')  style=Optimised  visibilities=8 + 2^11 + 2^18 + 2^19  flexible=off  slackgroup=0  augmented=0  version=20211007  advOptions=[]
  SynthesisInfo : DSPBAPrim/SynthesisInfo  primtype=synthinfo  nInputs=0  nOutputs=0  omode=Inherit via internal rule  otype=sfix(16)  scale=2^-15  rndmethod=Truncate  factor=1  satmethod=Symmetric  shift_vec=[0 1 2 -1]  value=99  inPortNames=[' '; ' ';]  outPortNames=[' ']  dspbaimage=dspba_prim_ctrl.jpg  text=fprintf('Style=%s', style);  style=Scheduled  visibilities=2^17+2^18+2^19+2^20+2^21+2^22+2^23+2^24  constraintPair=None  constraintRelation=>  constraintLimit=2  modelRefSign=+  modelRef=''  showSchedule=off  simulationMode=Use Global Value  resetMinimization=Conditional - On for ChannelIn/Out only  version=20220106
  data_out : Outport
  valid_out : Outport  Port=2
  ch_out : Outport  Port=3
  wires:
  Fallingedge/1(Out1) -> Loop/1
  Const2/1 -> Loop/2
  Const1/1 -> Loop/3
  Loop/1 -> Or/3
  ChannelIn/4 -> Or/1, SampleDelay/1, Fallingedge/1(In2)
  SampleDelay/1 -> Or/2
  ChannelIn/3 -> ChannelOut/3
  ch_in/1 -> ChannelIn/2
  ChannelIn/2 -> ChannelOut/2
  Or/1 -> Mux/1
  Mux/1 -> ChannelOut/1
  valid_in/1 -> ChannelIn/1
  ChannelIn/1 -> Mux/2
  ChannelOut/3 -> data_out/1
  Const/1 -> Mux/3
  ChannelOut/2 -> ch_out/1
  ChannelOut/1 -> valid_out/1
  flush_en/1 -> ChannelIn/4
  data_in/1 -> ChannelIn/3

== system Lib_LongPRACH/Longprach_C_M_plane/LongPRACH_core/DECIMATION1/stage4/Filt_DEC_by_2_stage4 ==
  din : Inport
  vin : Inport  Port=2
  cin : Inport  Port=3
  Complex to Real-Imag : ComplexToRealImag
  Const1 : DSPBAPrim/Const  primtype=const  nInputs=0  nOutputs=1  omode=Inherit via back propagation  otype=ufix(8)  scale=2^0  rndmethod=Unbiased  factor=1  satmethod=Symmetric  shift_vec=[0 1 2 -1]  value=deimator_shift  inPortNames=['+'; '+';]  outPortNames=[' ']  dspbaimage=dspba_prim.svg  text=fprintf('%s', num2str(value));  style=Optimised  visibilities=8 + 1024  floatPrecision=float32_m23  warnSaturation=on  version=20211007  SampleTime=inf
  Const6 : DSPBAPrim/Const  primtype=const  nInputs=0  nOutputs=1  omode=Inherit via back propagation  otype=ufix(8)  scale=2^0  rndmethod=Unbiased  factor=1  satmethod=Symmetric  shift_vec=[0 1 2 -1]  value=deimator_shift  inPortNames=['+'; '+';]  outPortNames=[' ']  dspbaimage=dspba_prim.svg  text=fprintf('%s', num2str(value));  style=Optimised  visibilities=8 + 1024  floatPrecision=float32_m23  warnSaturation=on  version=20211007  SampleTime=inf
  DecimatingFIR : DSPBAFilters/DecimatingFIR  nInputRate=prach.MaxSampleRate/(3*2*2)  decim=2  nchan=prach.no_of_chan  symmetry=Symmetrical  coef=b_decimator4  addr=MMoffset.HBcoef3  rwmode=Constant  nband=Use All Taps  exposebus=off  latency=98  version=20090407  recon=off  MM=[0,1,2,3,4,5,6,7,8,9,10,11,12,13,14,15]  resetrezero=off  sharecoef=auto  simulationMode=Standard
  DecimatingFIR1 : DSPBAFilters/DecimatingFIR  nInputRate=prach.MaxSampleRate/(3*2*2)  decim=2  nchan=prach.no_of_chan  symmetry=Symmetrical  coef=b_decimator4  addr=MMoffset.HBcoef3  rwmode=Constant  nband=Use All Taps  exposebus=off  latency=98  version=20090407  recon=off  MM=[0,1,2,3,4,5,6,7,8,9,10,11,12,13,14,15]  resetrezero=off  sharecoef=auto  simulationMode=Standard
  Real-Imag to Complex : RealImagToComplex
  Scale : DSPBABase/Scale  otype=sfix(16)  scale=2^-15  rndmethod=Biased  factor=decimator_gain4  satmethod=Symmetric  shift_vec=0  latency=5  simulationMode=Use Global Value  version=20130807
  Scale1 : DSPBABase/Scale  otype=sfix(16)  scale=2^-15  rndmethod=Biased  factor=decimator_gain4  satmethod=Symmetric  shift_vec=0  latency=5  simulationMode=Use Global Value  version=20130807
  Terminator{,1..3} (4 alike) : Terminator
  To Workspace3 : ToWorkspace  VariableName=dec_dout_stage4  SampleTime=-1
  To Workspace4 : ToWorkspace  VariableName=dec_vout_stage4  SampleTime=-1
  dout : Outport  VectorParamsAs1DForOutWhenUnconnected=off
  vout : Outport  Port=2  VectorParamsAs1DForOutWhenUnconnected=off
  cout : Outport  Port=3  VectorParamsAs1DForOutWhenUnconnected=off
  wires:
  DecimatingFIR/1 -> Scale/1
  Const6/1 -> Scale/4
  cin/1 -> DecimatingFIR1/3, DecimatingFIR/3
  Scale/4 -> Terminator/1
  DecimatingFIR/3 -> Scale/3
  vin/1 -> DecimatingFIR1/2, DecimatingFIR/2
  DecimatingFIR/2 -> Scale/2
  Scale/3 -> cout/1
  din/1 -> Complex to Real-Imag/1
  Complex to Real-Imag/1 -> DecimatingFIR/1
  Complex to Real-Imag/2 -> DecimatingFIR1/1
  DecimatingFIR1/1 -> Scale1/1
  DecimatingFIR1/3 -> Scale1/3
  Scale1/1 -> Real-Imag to Complex/2
  DecimatingFIR1/2 -> Scale1/2
  Const1/1 -> Scale1/4
  Scale1/4 -> Terminator1/1
  Scale/1 -> Real-Imag to Complex/1
  Scale1/2 -> Terminator2/1
  Scale1/3 -> Terminator3/1
  Scale/2 -> To Workspace4/1, vout/1
  Real-Imag to Complex/1 -> To Workspace3/1, dout/1

== system Lib_LongPRACH/Longprach_C_M_plane/LongPRACH_core/FFTShift/ChNoLatch/risingedge ==
  In2 : Inport
  And : DSPBAPrim/And  primtype=and  nInputs=2  nOutputs=1  omode=Inherit via internal rule  otype=sfix(16)  scale=2^-15  rndmethod=Unbiased  factor=1  satmethod=Symmetric  shift_vec=[0 1 2 -1]  value=0  inPortNames=[' '; ' '; ' '; ' '; ' '; ' '; ' '; ' '; ' '; ' '; ' '; ' '; ' '; ' '; ' '; ' '; ]  outPortNames=[' ']  dspbaimage=dspba_prim.svg  text=fprintf('&');  style=Optimised  visibilities=8+2  version=20211007
  Not : DSPBAPrim/Not  primtype=not  nInputs=1  nOutputs=1  omode=Inherit via internal rule  otype=sfix(16)  scale=2^-15  rndmethod=Unbiased  factor=1  satmethod=Symmetric  shift_vec=[0 1 2 -1]  value=0  inPortNames=[' '; ' ';]  outPortNames=[' ']  dspbaimage=dspba_prim.svg  text=fprintf('~');  style=Optimised  visibilities=8  version=20211007
  SampleDelay : DSPBAPrim/SampleDelay  primtype=sampdelay  nInputs=1  nOutputs=1  omode=Inherit via internal rule  otype=sfix(16)  scale=2^-15  rndmethod=Unbiased  factor=1  satmethod=Symmetric  shift_vec=[0 1 2 -1]  floatPrecision=float32_m23  value=1  inPortNames=[' '; ' ';]  outPortNames=[' ']  dspbaimage=dspba_prim.svg  text=dpoly(1, eye(1,value+1), 'z')  style=Optimised  visibilities=8 + 2^11 + 2^18 + 2^19  flexible=off  slackgroup=0  augmented=0  version=20211007  advOptions=[]
  Out1 : Outport
  wires:
  And/1 -> Out1/1
  In2/1 -> And/1, SampleDelay/1
  SampleDelay/1 -> Not/1
  Not/1 -> And/2

== system Lib_LongPRACH/Longprach_C_M_plane/LongPRACH_core/FFTShift/ChNoLatch/risingedge1 ==
  In2 : Inport
  And : DSPBAPrim/And  primtype=and  nInputs=2  nOutputs=1  omode=Inherit via internal rule  otype=sfix(16)  scale=2^-15  rndmethod=Unbiased  factor=1  satmethod=Symmetric  shift_vec=[0 1 2 -1]  value=0  inPortNames=[' '; ' '; ' '; ' '; ' '; ' '; ' '; ' '; ' '; ' '; ' '; ' '; ' '; ' '; ' '; ' '; ]  outPortNames=[' ']  dspbaimage=dspba_prim.svg  text=fprintf('&');  style=Optimised  visibilities=8+2  version=20211007
  Not : DSPBAPrim/Not  primtype=not  nInputs=1  nOutputs=1  omode=Inherit via internal rule  otype=sfix(16)  scale=2^-15  rndmethod=Unbiased  factor=1  satmethod=Symmetric  shift_vec=[0 1 2 -1]  value=0  inPortNames=[' '; ' ';]  outPortNames=[' ']  dspbaimage=dspba_prim.svg  text=fprintf('~');  style=Optimised  visibilities=8  version=20211007
  SampleDelay : DSPBAPrim/SampleDelay  primtype=sampdelay  nInputs=1  nOutputs=1  omode=Inherit via internal rule  otype=sfix(16)  scale=2^-15  rndmethod=Unbiased  factor=1  satmethod=Symmetric  shift_vec=[0 1 2 -1]  floatPrecision=float32_m23  value=1  inPortNames=[' '; ' ';]  outPortNames=[' ']  dspbaimage=dspba_prim.svg  text=dpoly(1, eye(1,value+1), 'z')  style=Optimised  visibilities=8 + 2^11 + 2^18 + 2^19  flexible=off  slackgroup=0  augmented=0  version=20211007  advOptions=[]
  Out1 : Outport
  wires:
  And/1 -> Out1/1
  In2/1 -> And/1, SampleDelay/1
  SampleDelay/1 -> Not/1
  Not/1 -> And/2

== system Lib_LongPRACH/Longprach_C_M_plane/LongPRACH_core/FFTShift/Mem_rd_wr/Mem_rd_control ==
  wba : Inport
  BitCombine : DSPBAPrim/BitCombine  primtype=bitcombine  nInputs=2  nOutputs=1  omode=Inherit via internal rule  otype=sfix(16)  scale=2^-15  rndmethod=Unbiased  factor=1  satmethod=Symmetric  shift_vec=[0 1 2 -1]  value=0  inPortNames=['l'; 'h';]  outPortNames=[' ']  dspbaimage=dspba_prim.svg  text=fprintf('[h,l]');  style=Optimised  visibilities=8+2  version=20211007
  Const1 : DSPBAPrim/Const  primtype=const  nInputs=0  nOutputs=1  omode=boolean  otype=fixdt(0,2,0)  scale=0  rndmethod=Unbiased  factor=1  satmethod=Symmetric  shift_vec=[0 1 2 -1]  value=1  inPortNames=['+'; '+';]  outPortNames=[' ']  dspbaimage=dspba_prim.svg  text=fprintf('%s', num2str(value));  style=Optimised  visibilities=8 + 1024  floatPrecision=float32_m23  warnSaturation=on  version=20211007  SampleTime=inf
  Const2 : DSPBAPrim/Const  primtype=const  nInputs=0  nOutputs=1  omode=Inherit via internal rule  otype=fixdt(0,10,0)  scale=0  rndmethod=Unbiased  factor=1  satmethod=Symmetric  shift_vec=[0 1 2 -1]  value=1024  inPortNames=['+'; '+';]  outPortNames=[' ']  dspbaimage=dspba_prim.svg  text=fprintf('%s', num2str(value));  style=Optimised  visibilities=8 + 1024  floatPrecision=float32_m23  warnSaturation=on  version=20211007  SampleTime=inf
  Convert : DSPBAPrim/Convert  primtype=convert  nInputs=1  nOutputs=1  omode=Specify via dialog  otype=fixdt(0,10,0)  scale=0  rndmethod=Unbiased  factor=1  satmethod=None  shift_vec=[0 1 2 -1]  value=round([0:255]/17)  inPortNames=[' '; ' ';]  outPortNames=[' '; 'c']  dspbaimage=dspba_prim_wide.svg  text=fprintf('convert');  style=Optimised  visibilities=8+64+256+2^17  clipdetect=off  floatPrecision=float32_m23  advOptions=[]  version=20211007
  EdgeDetect : Subsystem
  FFT_shiftAddrMap : Subsystem
  Loop : DSPBAPrim/Loop  primtype=loop  nInputs=3  nOutputs=4  omode=Inherit via internal rule  otype=sfix(16)  scale=2^-15  rndmethod=Unbiased  factor=1  satmethod=Symmetric  shift_vec=[0 1 2 -1]  value=[zeros(16, 1)]  inPortNames=['g'; 'c'; 'e']  outPortNames=['v'; 'q'; 'f'; 'l']  dspbaimage=dspba_prim_tall.svg  text=fprintf('loop');  style=Optimised  visibilities=0  version=20211007
  Not : DSPBAPrim/Not  primtype=not  nInputs=1  nOutputs=1  omode=Inherit via internal rule  otype=sfix(16)  scale=2^-15  rndmethod=Unbiased  factor=1  satmethod=Symmetric  shift_vec=[0 1 2 -1]  value=0  inPortNames=[' '; ' ';]  outPortNames=[' ']  dspbaimage=dspba_prim.svg  text=fprintf('~');  style=Optimised  visibilities=8  version=20211007
  rd_addr_final : Outport
  validout : Outport  Port=2
  wires:
  Loop/2 -> Convert/1
  Convert/1 -> FFT_shiftAddrMap/1(In1)
  FFT_shiftAddrMap/1(Out1) -> BitCombine/1
  Loop/1 -> validout/1
  Not/1 -> BitCombine/2  "rba"
  BitCombine/1 -> rd_addr_final/1
  EdgeDetect/1(Out1) -> Loop/1
  wba/1 -> EdgeDetect/1(In1), Not/1
  Const2/1 -> Loop/2
  Const1/1 -> Loop/3

== system Lib_LongPRACH/Longprach_C_M_plane/LongPRACH_core/FFTShift/Mem_rd_wr/Mem_wr_control ==
  valid : Inport
  Wr_addr_gen : Subsystem
  wr_addr_final : Outport
  we : Outport  Port=2
  wba : Outport  Port=3
  wires:
  Wr_addr_gen/1(wba) -> wba/1
  Wr_addr_gen/3(we) -> we/1
  Wr_addr_gen/2(wr_addr) -> wr_addr_final/1
  valid/1 -> Wr_addr_gen/1(valid)

== system Lib_LongPRACH/Longprach_C_M_plane/LongPRACH_core/S2B_FFT/S2B/S2B_control ==
  valid : Inport
  ch_no_in : Inport  Port=2
  resetin : Inport  Port=3
  Mem_rd_control : Subsystem
  Mem_wr_control : Subsystem
  Wr_addr_final : Outport
  We : Outport  Port=2
  rd_addr_final : Outport  Port=3
  rd_validout : Outport  Port=4
  ch_no : Outport  Port=5
  wires:
  Mem_rd_control/3(ch_no) -> ch_no/1
  Mem_rd_control/2(validout) -> rd_validout/1
  Mem_rd_control/1(rd_addr_final) -> rd_addr_final/1
  Mem_wr_control/3(wba) -> Mem_rd_control/1(wba)
  Mem_wr_control/2(we) -> We/1
  Mem_wr_control/1(wr_addr_final) -> Wr_addr_final/1
  valid/1 -> Mem_wr_control/1(valid)
  ch_no_in/1 -> Mem_wr_control/2(ch_no)
  resetin/1 -> Mem_wr_control/3(resetin)

== system Lib_LongPRACH/Longprach_C_M_plane/LongPRACH_core/SYM_SELECT/Zero_insertion/Zeropad_front ==
  valid_in : Inport
  chin : Inport  Port=2
  datain : Inport  Port=3
  And : DSPBAPrim/And  primtype=and  nInputs=2  nOutputs=1  omode=Inherit via internal rule  otype=sfix(16)  scale=2^-15  rndmethod=Unbiased  factor=1  satmethod=Symmetric  shift_vec=[0 1 2 -1]  value=0  inPortNames=[' '; ' '; ' '; ' '; ' '; ' '; ' '; ' '; ' '; ' '; ' '; ' '; ' '; ' '; ' '; ' '; ]  outPortNames=[' ']  dspbaimage=dspba_prim.svg  text=fprintf('&');  style=Optimised  visibilities=8+2  version=20211007
  Const3 : DSPBAPrim/Const  primtype=const  nInputs=0  nOutputs=1  omode=Inherit via internal rule  otype=sfix(16)  scale=2^-15  rndmethod=Unbiased  factor=1  satmethod=Symmetric  shift_vec=[0 1 2 -1]  value=0  inPortNames=['+'; '+';]  outPortNames=[' ']  dspbaimage=dspba_prim.svg  text=fprintf('%s', num2str(value));  style=Optimised  visibilities=8 + 1024 + 2^18 + 2^20  floatPrecision=float32_m23  warnSaturation=on  version=20211007  SampleTime=inf
  Mux1 : DSPBAPrim/Mux  primtype=mux  nInputs=evalAionMaskParam(gcb,'value',1)+1  nOutputs=1  omode=Inherit via internal rule  otype=sfix(16)  scale=2^-15  rndmethod=Unbiased  factor=1  satmethod=Symmetric  shift_vec=[0 1 2 -1]  value=2  inPortNames=['s '; 'd0'; 'd1'; 'd2'; 'd3'; 'd4'; 'd5'; 'd6'; 'd7'; 'd8'; 'd9';]  outPortNames=[' ']  dspbaimage=dspba_prim_tall.svg  text=fprintf('%s', primtype);  style=Optimised  visibilities=1032  version=20211007
  Not : DSPBAPrim/Not  primtype=not  nInputs=1  nOutputs=1  omode=Inherit via internal rule  otype=sfix(16)  scale=2^-15  rndmethod=Unbiased  factor=1  satmethod=Symmetric  shift_vec=[0 1 2 -1]  value=0  inPortNames=[' '; ' ';]  outPortNames=[' ']  dspbaimage=dspba_prim.svg  text=fprintf('~');  style=Optimised  visibilities=8  version=20211007
  Or : DSPBAPrim/Or  primtype=or  nInputs=2  nOutputs=1  omode=Inherit via internal rule  otype=sfix(16)  scale=2^-15  rndmethod=Unbiased  factor=1  satmethod=Symmetric  shift_vec=[0 1 2 -1]  value=0  inPortNames=[' '; ' '; ' '; ' '; ' '; ' '; ' '; ' '; ' '; ' '; ' '; ' '; ' '; ' '; ' '; ' '; ]  outPortNames=[' ']  dspbaimage=dspba_prim.svg  text=fprintf('|');  style=Optimised  visibilities=8+2  version=20211007
  SampleDelay1 : DSPBAPrim/SampleDelay  primtype=sampdelay  nInputs=1  nOutputs=1  omode=Inherit via internal rule  otype=sfix(16)  scale=2^-15  rndmethod=Unbiased  factor=1  satmethod=Symmetric  shift_vec=[0 1 2 -1]  floatPrecision=float32_m23  value=ZeroPadFront  inPortNames=[' '; ' ';]  outPortNames=[' ']  dspbaimage=dspba_prim.svg  text=dpoly(1, eye(1,value+1), 'z')  style=Optimised  visibilities=8 + 2^11 + 2^18 + 2^19  flexible=off  slackgroup=0  augmented=0  version=20211007  advOptions=[]
  SampleDelay2 : DSPBAPrim/SampleDelay  primtype=sampdelay  nInputs=1  nOutputs=1  omode=Inherit via internal rule  otype=sfix(16)  scale=2^-15  rndmethod=Unbiased  factor=1  satmethod=Symmetric  shift_vec=[0 1 2 -1]  floatPrecision=float32_m23  value=ZeroPadFront  inPortNames=[' '; ' ';]  outPortNames=[' ']  dspbaimage=dspba_prim.svg  text=dpoly(1, eye(1,value+1), 'z')  style=Optimised  visibilities=8 + 2^11 + 2^18 + 2^19  flexible=off  slackgroup=0  augmented=0  version=20211007  advOptions=[]
  valid_out : Outport
  "chout " : Outport  Port=2
  dataout : Outport  Port=3
  wires:
  And/1 -> Mux1/1
  valid_in/1 -> SampleDelay2/1, Or/1, And/1
  SampleDelay2/1 -> Or/2, Not/1
  chin/1 -> "chout "/1
  SampleDelay1/1 -> Mux1/2
  datain/1 -> SampleDelay1/1
  Or/1 -> valid_out/1
  Not/1 -> And/2
  Mux1/1 -> dataout/1
  Const3/1 -> Mux1/3
